simulink model "mExternalMfile"  (Simulink 9.0)
settings: Solver=FixedStepDiscrete  StartTime=0.0  StopTime=10.0  FixedStep=0.2  RelTol=1e-3  EnableMultiTasking=on
libraries: mExternalMlib x1
settings Model: Creator=dalparsl  LastModifiedBy=apuvvala
settings DataIOCC: LimitDataPoints=on  SignalLoggingSaveFormat=ModelDataLogs
settings OptimizationCC: ExpressionDepthLimit=2147483647  InitFltsAndDblsToZero=on
settings DebuggingCC: SolverPrmCheckMsg=warning  FcnCallInpInsideContextMsg=warning  StateNameClashWarn=warning
settings SFSimCC: SimParseCustomCode=off
settings GRTTargetCC: CombineOutputUpdateFcns=off  GRTInterface=on
settings ConfigComp: CovEnable=on  RecordCoverage=on  CovMetricSettings=dcmtrzwe  CovCumulativeReport=on  CovModelRefEnable=on  CovExternalEMLEnable=on

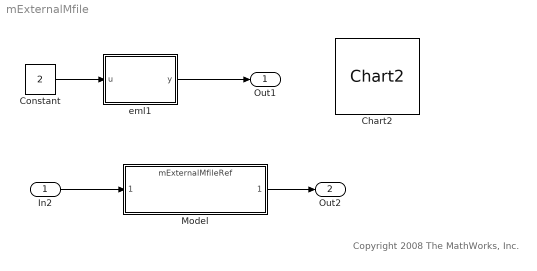
== system mExternalMfile ==
  note: Copyright 2008 The MathWorks, Inc.
  In2 : Inport  OutDataTypeStr=double
  Chart2 : mExternalMlib/Chart2
  Constant : Constant  Value=2
  Model : ModelReference  ModelNameDialog=mExternalMfileRef  SimulationMode=Normal  ModelReferenceVersion=1.15
  eml1 : MATLAB Function  TreatAsAtomicUnit=on
  Out1 : Outport
  Out2 : Outport  Port=2
  wires:
  Constant/1 -> eml1/1(u)
  eml1/1(y) -> Out1/1
  In2/1 -> Model/1
  Model/1 -> Out2/1

== matlab function eml1 ==
  data: u input double; y output double
function y = fcn(u)
% This block supports the Embedded MATLAB subset.
% See the help menu for details. 
a = externalmfile(u);
b = externalmfile1(u+7);
c = externalmfile2(u);
y =a+b+2 +c;
